simulink model "teleop_delay_system"  (R2025b)
settings: Solver=ode4  StartTime=0.0  StopTime=10  FixedStep=0.01  RelTol=1e-3
model workspace (MAT data in the model file):
  delay_s = 0.1
  sample_period_s = 0.05
  time_constant_s = 0.2
settings Model: Creator=miyut  LastModifiedBy=miyut
settings DataIOCC: SignalLogging=off

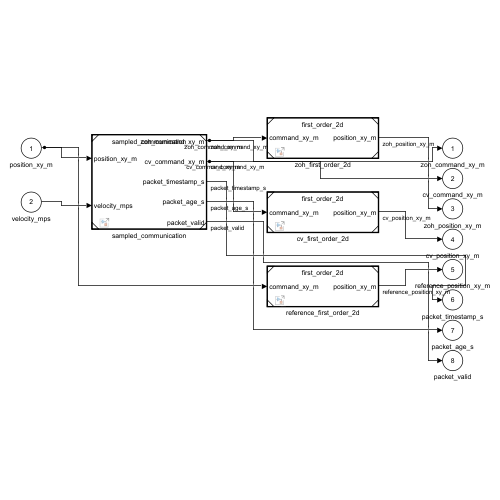
[thumbnail: Simulink's stored preview of the top-level diagram]
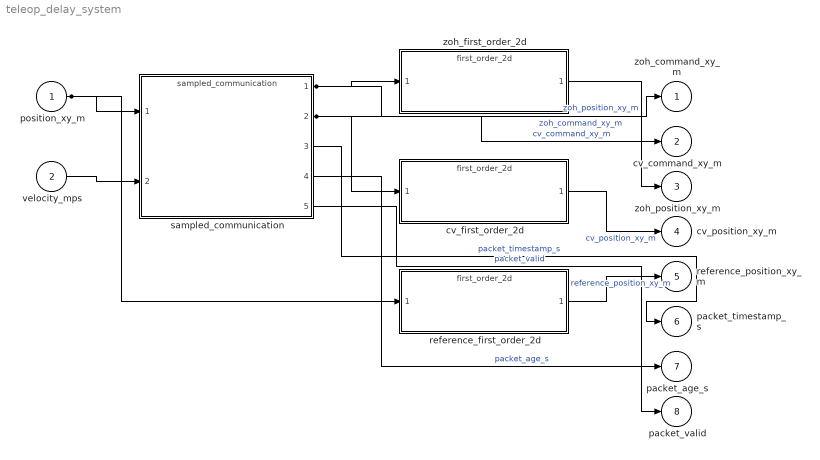
== system teleop_delay_system ==
  position_xy_m : Inport  OutDataTypeStr=double  Unit=m  PortDimensions=2
  velocity_mps : Inport  Port=2  OutDataTypeStr=double  Unit=m/s  PortDimensions=2
  cv_first_order_2d : ModelReference  ModelNameDialog=first_order_2d  ParameterArgumentNames=time_constant_s  ParameterArgumentValues=time_constant_s  UsingDefaultArgumentValue=0  SimulationMode=Normal  ModelReferenceVersion=1.1
  reference_first_order_2d : ModelReference  ModelNameDialog=first_order_2d  ParameterArgumentNames=time_constant_s  ParameterArgumentValues=time_constant_s  UsingDefaultArgumentValue=0  SimulationMode=Normal  ModelReferenceVersion=1.1
  sampled_communication : ModelReference  ModelNameDialog=sampled_communication  UsingDefaultArgumentValue=0,0  SimulationMode=Normal  ModelReferenceVersion=1.1
  zoh_first_order_2d : ModelReference  ModelNameDialog=first_order_2d  ParameterArgumentNames=time_constant_s  ParameterArgumentValues=time_constant_s  UsingDefaultArgumentValue=0  SimulationMode=Normal  ModelReferenceVersion=1.1
  zoh_command_xy_m : Outport  OutDataTypeStr=double  Unit=m  PortDimensions=2
  cv_command_xy_m : Outport  Port=2  OutDataTypeStr=double  Unit=m  PortDimensions=2
  zoh_position_xy_m : Outport  Port=3  OutDataTypeStr=double  Unit=m  PortDimensions=2
  cv_position_xy_m : Outport  Port=4  OutDataTypeStr=double  Unit=m  PortDimensions=2
  reference_position_xy_m : Outport  Port=5  OutDataTypeStr=double  Unit=m  PortDimensions=2
  packet_timestamp_s : Outport  Port=6  OutDataTypeStr=double  Unit=s  PortDimensions=1
  packet_age_s : Outport  Port=7  OutDataTypeStr=double  Unit=s  PortDimensions=1
  packet_valid : Outport  Port=8  OutDataTypeStr=boolean  PortDimensions=1
  wires:
  position_xy_m/1 -> sampled_communication/1, reference_first_order_2d/1
  velocity_mps/1 -> sampled_communication/2
  sampled_communication/1 -> zoh_first_order_2d/1, zoh_command_xy_m/1  "zoh_command_xy_m"
  sampled_communication/2 -> cv_first_order_2d/1, cv_command_xy_m/1  "cv_command_xy_m"
  zoh_first_order_2d/1 -> zoh_position_xy_m/1  "zoh_position_xy_m"
  cv_first_order_2d/1 -> cv_position_xy_m/1  "cv_position_xy_m"
  reference_first_order_2d/1 -> reference_position_xy_m/1  "reference_position_xy_m"
  sampled_communication/3 -> packet_timestamp_s/1  "packet_timestamp_s"
  sampled_communication/4 -> packet_age_s/1  "packet_age_s"
  sampled_communication/5 -> packet_valid/1  "packet_valid"
